simulink library "mconversion12aLib2"  (Simulink 6.0)
settings: Solver=ode45  StartTime=0.0  StopTime=10.0  RelTol=1e-3
libraries: mconversion12aLib1 x1
settings Model: Creator=mshakeri  LastModifiedBy=awarlock  ExtModeAutoUpdateStatusClock=off
settings DebuggingCC: CheckExecutionContextPreStartOutputMsg=on  CheckExecutionContextRuntimeOutputMsg=on
settings SFSimCC: SFSimApplyToAllLibs=on  SFSimBuildMode=Incremental

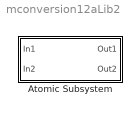
== system mconversion12aLib2 ==
  Atomic Subsystem : Subsystem  TreatAsAtomicUnit=on  PropExecContextAcrossSSBoundary=on

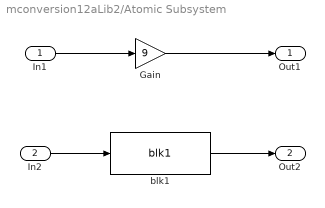
== system mconversion12aLib2/Atomic Subsystem ==
  In1 : Inport  LatchInput=off
  In2 : Inport  Port=2  LatchInput=off
  Gain : Gain  Gain=9
  blk1 : mconversion12aLib1/blk1
  Out1 : Outport
  Out2 : Outport  Port=2
  wires:
  blk1/1 -> Out2/1
  In2/1 -> blk1/1
  Gain/1 -> Out1/1
  In1/1 -> Gain/1
